simulink model "part_2"  (R2025b)
settings: Solver=VariableStepAuto  StartTime=0.0  StopTime=10.0  RelTol=1e-3
settings Model: SimulationMode=accelerator  Creator=Ultor  LastModifiedBy=Ultor

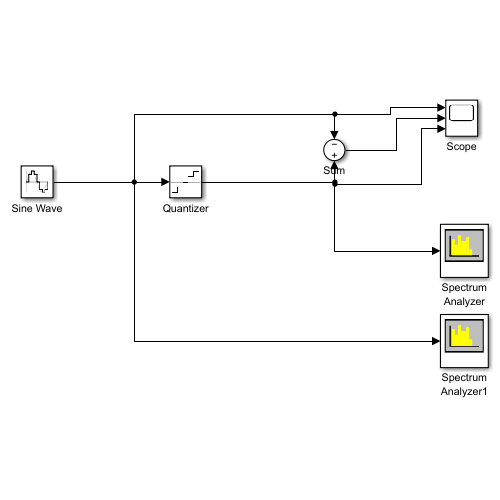
[thumbnail: Simulink's stored preview of the top-level diagram]
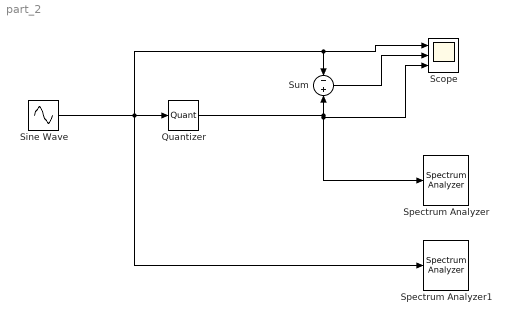
== system part_2 ==
  Quantizer : Quantizer  QuantizationInterval=16
  Scope : Scope  NumInputPorts=3
      settings: ActiveDisplayYMinimum=-20  ActiveDisplayYMaximum=20
  Sine Wave : Sin  Amplitude=11  Frequency=21*pi*2  SampleTime=1/1000
  Spectrum Analyzer : SpectrumAnalyzer  WindowPosition=[962.000000,566.000000,958.000000,484.000000,]  Visible=on  ScopeFrameLocation=window  PlotAsTwoSidedSpectrum=off  WindowInvariantSamplesPerUpdate=on  YLimits=[-53.405 59.0713]  SelectedToolstripTab=spectrumAnalyzerToolstrip.spectrumTab
  Spectrum Analyzer1 : SpectrumAnalyzer  WindowPosition=[962.000000,50.000000,958.000000,484.000000,]  Visible=on  ScopeFrameLocation=window  SpectrumType=Power density  PlotAsTwoSidedSpectrum=off  WindowInvariantSamplesPerUpdate=on  FrequencySpan=Start and stop frequencies  StartFrequency=0  StopFrequency=63  SpectrumUnits=dBm/Hz  YLimits=[-41.9722 64.1665]  SelectedToolstripTab=spectrumAnalyzerToolstrip.spectrumTab
  Sum : Sum  Inputs=-+
  wires:
  Sine Wave/1 -> Spectrum Analyzer1/1, Scope/1, Sum/1, Quantizer/1
  Quantizer/1 -> Scope/3, Spectrum Analyzer/1, Sum/2
  Sum/1 -> Scope/2
